simulink model "ejemplo2"  (R2013b)
settings: Solver=ode45  StartTime=0.0  StopTime=10.0  RelTol=1e-3
settings Model: Creator=user  LastModifiedBy=user
settings DataIOCC: SaveFormat=StructureWithTime  SaveState=on

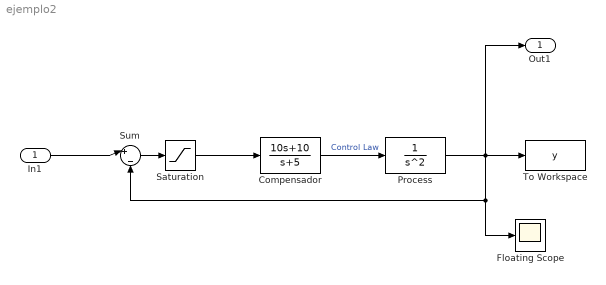
== system ejemplo2 ==
  In1 : Inport
  Compensador : TransferFcn  Numerator=[10 10]  Denominator=[1 5]
  Floating Scope : Scope
  Process : TransferFcn  Denominator=[1 0 0]
  Saturation : Saturate  UpperLimit=1  LowerLimit=-1
  Sum : Sum  Inputs=|+|-
  To Workspace : ToWorkspace  VariableName=y  SampleTime=-1  SaveFormat=Timeseries
  Out1 : Outport
  wires:
  Compensador/1 -> Process/1  "Control Law"
  Process/1 -> Floating Scope/1, Sum/2, Out1/1, To Workspace/1
  In1/1 -> Sum/1
  Saturation/1 -> Compensador/1
  Sum/1 -> Saturation/1
